simulink model "modelo_LTI"  (R2018a)
settings: Solver=VariableStepAuto  StartTime=0.0  StopTime=10.0  RelTol=1e-3
values from neighbouring files (symbols this model uses):
  b_eq = b_m + b_l/r^2    (= 1.5e-05)    [proyecto_global_integrador.m]
  J_eq = J_m + J_l/r^2    (= 5.65099476805e-06)    [proyecto_global_integrador.m]
  L_q = 5.8e-3    (= 0.0058)    [proyecto_global_integrador.m]
  lambda_m = 0.01546    [proyecto_global_integrador.m]
  P_p = 3    [proyecto_global_integrador.m]
  r = 314.3008    [proyecto_global_integrador.m]
  R_s = 1.02    [polos_choreo_no_se_puede_robar_mas_con_esto.m]    (also in proyecto_global_integrador.m)
settings Model: Creator=gabrielq  LastModifiedBy=gabrielq

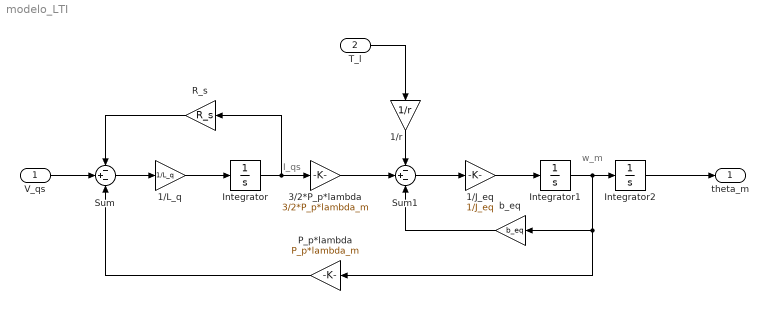
== system modelo_LTI ==
  note: I_qs
  note: w_m
  V_qs : Inport
  T_l : Inport  Port=2
  1/J_eq : Gain  Gain=1/J_eq
  1/L_q : Gain  Gain=1/L_q
  "1/r " : Gain  Gain=1/r
  3/2*P_p*lambda : Gain  Gain=3/2*P_p*lambda_m
  Integrator : Integrator
  Integrator1 : Integrator
  Integrator2 : Integrator
  P_p*lambda : Gain  Gain=P_p*lambda_m
  R_s : Gain  Gain=R_s
  Sum : Sum  Inputs=-+-
  Sum1 : Sum  Inputs=-+-
  b_eq : Gain  Gain=b_eq
  theta_m : Outport
  wires:
  V_qs/1 -> Sum/2
  R_s/1 -> Sum/1
  1/L_q/1 -> Integrator/1
  Integrator/1 -> R_s/1, 3/2*P_p*lambda/1
  3/2*P_p*lambda/1 -> Sum1/2
  P_p*lambda/1 -> Sum/3
  Sum/1 -> 1/L_q/1
  Sum1/1 -> 1/J_eq/1
  1/J_eq/1 -> Integrator1/1
  T_l/1 -> "1/r "/1
  "1/r "/1 -> Sum1/1
  b_eq/1 -> Sum1/3
  Integrator1/1 -> P_p*lambda/1, b_eq/1, Integrator2/1
  Integrator2/1 -> theta_m/1
